simulink model "fxpdemo_min_max_optimization"  (Simulink 7.6)
settings: Solver=FixedStepDiscrete  StartTime=0.0  StopTime=1  FixedStep=1  RelTol=1e-3
libraries: rtwdemowidgets x1
Description:
  | Fixed-Point Optimizations Using Specified Minimum and Maximum Values
  | 
  | This model shows fixed-point optimizations in generated code using minimum and maximum values that you specify in the model.
settings Model: Creator=The MathWorks Inc.  ExtModeAutoUpdateStatusClock=off
settings DataIOCC: LimitDataPoints=off  SaveFormat=Structure  SaveOutput=off  SaveTime=off
settings OptimizationCC: InlineParams=on  UseIntDivNetSlope=on  InlineInvariantSignals=on  EnhancedBackFolding=on  BooleansAsBitfields=on  PassReuseOutputArgsAs=Individual arguments  StateBitsets=on  DataBitsets=on  UseTempVars=on  ZeroExternalMemoryAtStartup=off  ZeroInternalMemoryAtStartup=off  EfficientFloat2IntCast=on  OptimizeModelRefInitCode=on  LifeSpan=1
settings DebuggingCC: SaveWithParameterizedLinksMsg=none  IntegerOverflowMsg=none  FcnCallInpInsideContextMsg=Enable All  UniqueDataStoreMsg=error  AssertControl=DisableAll  StrictBusMsg=Warning
settings HardwareCC: ProdIntDivRoundTo=Zero  ProdEndianess=LittleEndian  ProdHWDeviceType=Generic->32-bit Embedded Processor  TargetEndianess=LittleEndian  TargetHWDeviceType=MATLAB Host
settings RTWCC: SystemTargetFile=ert.tlc  GenCodeOnly=on  TemplateMakefile=ert_default_tmf  Description=Real-Time Workshop Embedded Coder  GenerateReport=on  RTWVerbose=off  ProcessScript=ert_make_rtw_hook  IncludeHyperlinkInReport=on  LaunchReport=on  GenerateTraceInfo=on  GenerateTraceReport=on  GenerateTraceReportSl=on  GenerateTraceReportSf=on  GenerateTraceReportEml=on
settings CodeAppCC: ForceParamTrailComments=on  IgnoreCustomStorageClasses=off  IgnoreTestpoints=on  SimulinkDataObjDesc=on  CustomSymbolStrGlobalVar=rt$N$M  CustomSymbolStrType=$N$M  CustomSymbolStrFcn=$N$M$F  CustomSymbolStrMacro=$N$M  InsertBlockDesc=on
settings ERTTargetCC: MultiwordLength=2048  GenerateSampleERTMain=on  IncludeMdlTerminateFcn=off  CombineSignalStateStructs=on  SupportNonFinite=off  SupportComplex=off  PurelyIntegerCode=on  InlinedParameterPlacement=NonHierarchical  ERTCustomFileTemplate=example_file_process.tlc  ERTFilePackagingFormat=CompactWithDataFile  ConvertIfToSwitch=off

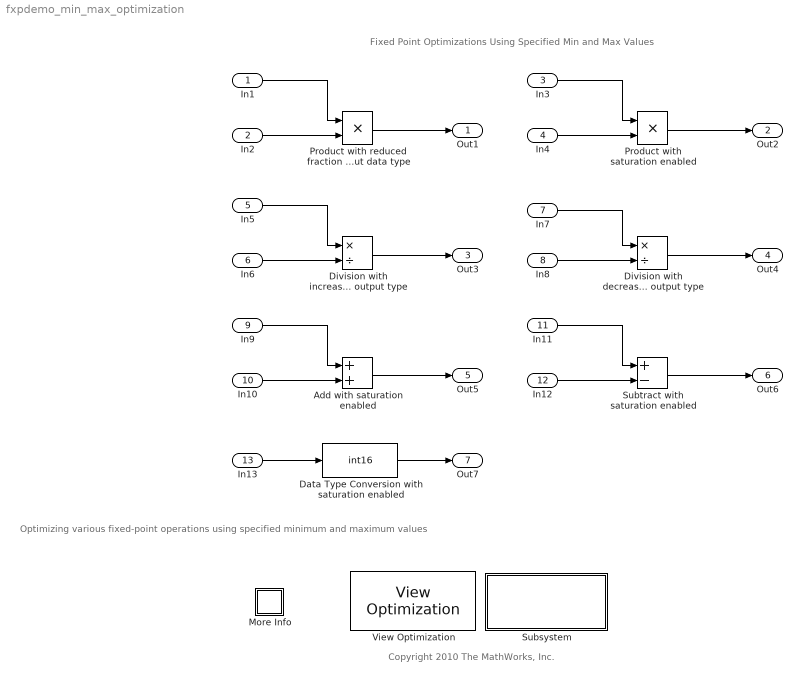
== system fxpdemo_min_max_optimization ==
  note: Copyright 2010 The MathWorks, Inc.
  note: Optimizing various fixed-point operations using specified minimum and maximum values
  note: Fixed Point Optimizations Using Specified Min and Max Values
  In1 : Inport  OutMin=1  OutMax=100  OutDataTypeStr=fixdt(0,32,10)  PortDimensions=1  SampleTime=1
      settings: AttributesFormatString=Min=%<OutMin>\nMax=%<OutMax>
  In2 : Inport  Port=2  OutMin=1  OutMax=100  OutDataTypeStr=uint32  PortDimensions=1  SampleTime=1
      settings: AttributesFormatString=Min=%<OutMin>\nMax=%<OutMax>
  In3 : Inport  Port=3  OutMin=1  OutMax=100  OutDataTypeStr=uint32  PortDimensions=1  SampleTime=1
      settings: AttributesFormatString=Min=%<OutMin>\nMax=%<OutMax>
  In4 : Inport  Port=4  OutMin=1  OutMax=100  OutDataTypeStr=uint32  PortDimensions=1  SampleTime=1
      settings: AttributesFormatString=Min=%<OutMin>\nMax=%<OutMax>
  In5 : Inport  Port=5  OutMin=1  OutMax=100  OutDataTypeStr=uint16  PortDimensions=1  SampleTime=1
      settings: AttributesFormatString=Min=%<OutMin>\nMax=%<OutMax>
  In6 : Inport  Port=6  OutDataTypeStr=uint16  PortDimensions=1  SampleTime=1
  In7 : Inport  Port=7  OutDataTypeStr=uint16  PortDimensions=1  SampleTime=1
  In8 : Inport  Port=8  OutMin=1  OutMax=100  OutDataTypeStr=uint16  PortDimensions=1  SampleTime=1
      settings: AttributesFormatString=Min=%<OutMin>\nMax=%<OutMax>
  In9 : Inport  Port=9  OutMin=-10  OutMax=10  OutDataTypeStr=int16  PortDimensions=1  SampleTime=1
      settings: AttributesFormatString=Min=%<OutMin>\nMax=%<OutMax>
  In10 : Inport  Port=10  OutMin=-10  OutMax=10  OutDataTypeStr=int16  PortDimensions=1  SampleTime=1
      settings: AttributesFormatString=Min=%<OutMin>\nMax=%<OutMax>
  In11 : Inport  Port=11  OutMin=0  OutMax=10  OutDataTypeStr=int16  PortDimensions=1  SampleTime=1
      settings: AttributesFormatString=Min=%<OutMin>\nMax=%<OutMax>
  In12 : Inport  Port=12  OutMin=0  OutMax=10  OutDataTypeStr=int16  PortDimensions=1  SampleTime=1
      settings: AttributesFormatString=Min=%<OutMin>\nMax=%<OutMax>
  In13 : Inport  Port=13  OutMin=-75  OutMax=100  OutDataTypeStr=int32  PortDimensions=1  SampleTime=1
      settings: AttributesFormatString=Min=%<OutMin>\nMax=%<OutMax>
  Add with saturation enabled : Sum  AccumDataTypeStr=int16  OutDataTypeStr=int16  SaturateOnIntegerOverflow=on
  Data Type Conversion with saturation enabled : DataTypeConversion  OutDataTypeStr=int16  SaturateOnIntegerOverflow=on
  Division with decreased fraction length output type : Product  Inputs=*/  OutDataTypeStr=fixdt(0,32,-17)  RndMeth=Simplest
  Division with increased fraction length output type : Product  Inputs=*/  OutDataTypeStr=fixdt(0,32,17)  RndMeth=Simplest
  More Info : Subsystem
      settings: OpenFcn=showdemo(sprintf('%s%s', bdroot(gcs), '_script'))
      mask Display: disp('?')
  Product with saturation enabled : Product  Inputs=**  OutDataTypeStr=uint32  SaturateOnIntegerOverflow=on  RndMeth=Zero
  Product with reduced fraction length output data type : Product  Inputs=**  OutDataTypeStr=uint32  RndMeth=Zero
  Subsystem : Subsystem
      settings: OpenFcn=rtwbuilddemomodel(bdroot);
      mask Display: disp('Generate Code\n(double-click)')
  Subtract with saturation enabled : Sum  Inputs=+-  AccumDataTypeStr=int16  OutDataTypeStr=int16  SaturateOnIntegerOverflow=on
  View Optimization : rtwdemowidgets/View Optimization  SystemSampleTime=-1
  Out1 : Outport
  Out2 : Outport  Port=2
  Out3 : Outport  Port=3
  Out4 : Outport  Port=4
  Out5 : Outport  Port=5
  Out6 : Outport  Port=6
  Out7 : Outport  Port=7
  wires:
  Division with increased fraction length output type/1 -> Out3/1
  In5/1 -> Division with increased fraction length output type/1
  In6/1 -> Division with increased fraction length output type/2
  Product with saturation enabled/1 -> Out2/1
  In3/1 -> Product with saturation enabled/1
  In4/1 -> Product with saturation enabled/2
  Division with decreased fraction length output type/1 -> Out4/1
  In7/1 -> Division with decreased fraction length output type/1
  In8/1 -> Division with decreased fraction length output type/2
  In9/1 -> Add with saturation enabled/1
  In10/1 -> Add with saturation enabled/2
  Add with saturation enabled/1 -> Out5/1
  In11/1 -> Subtract with saturation enabled/1
  In12/1 -> Subtract with saturation enabled/2
  Subtract with saturation enabled/1 -> Out6/1
  In13/1 -> Data Type Conversion with saturation enabled/1
  Data Type Conversion with saturation enabled/1 -> Out7/1
  In2/1 -> Product with reduced fraction length output data type/2
  In1/1 -> Product with reduced fraction length output data type/1
  Product with reduced fraction length output data type/1 -> Out1/1

== system fxpdemo_min_max_optimization/More Info ==

== system fxpdemo_min_max_optimization/Subsystem ==
